simulink model "magnetorquer"  (R2019b)
settings: Solver=VariableStepAuto  StartTime=0.0  StopTime=10.0  RelTol=1e-3
libraries: vrlib x1
settings Model: Creator=Florian  LastModifiedBy=robin

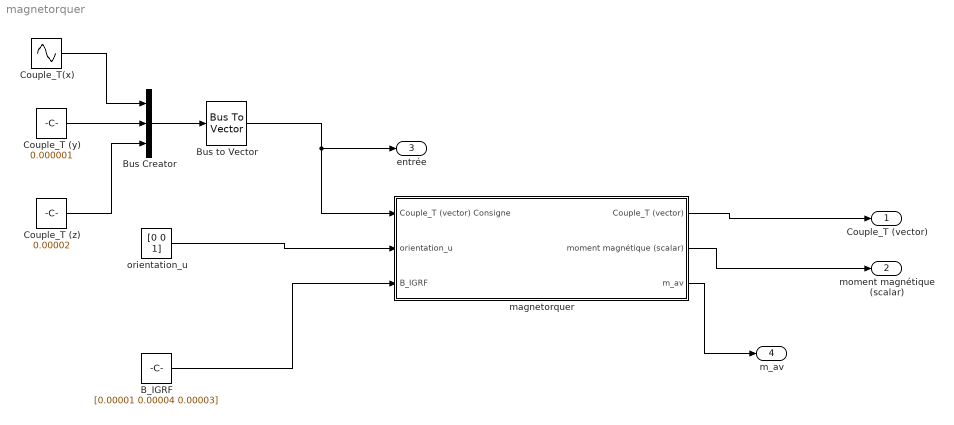
== system magnetorquer ==
  B_IGRF : Constant  Value=[0.00001 0.00004 0.00003]
  Bus Creator : BusCreator  Inputs=3
  Bus to Vector : BusToVector
  Couple_T (y) : Constant  Value=0.000001
  "Couple_T (z) " : Constant  Value=0.00002
  Couple_T(x) : Sin  Amplitude=0.00005  Phase=0.2  SampleTime=0
  magnetorquer : Subsystem
  "orientation_u " : Constant  Value=[0 0 1]
  "Couple_T (vector) " : Outport
  moment magnétique (scalar) : Outport  Port=2
  entrée : Outport  Port=3
  m_av : Outport  Port=4
  wires:
  Bus to Vector/1 -> entrée/1, magnetorquer/1(Couple_T (vector) Consigne)
  "orientation_u "/1 -> magnetorquer/2(orientation_u)
  B_IGRF/1 -> magnetorquer/3(B_IGRF)
  magnetorquer/1("Couple_T (vector) ") -> "Couple_T (vector) "/1
  magnetorquer/2(moment magnétique (scalar)) -> moment magnétique (scalar)/1
  Bus Creator/1 -> Bus to Vector/1
  Couple_T (y)/1 -> Bus Creator/2
  "Couple_T (z) "/1 -> Bus Creator/3
  Couple_T(x)/1 -> Bus Creator/1
  magnetorquer/3(m_av) -> m_av/1

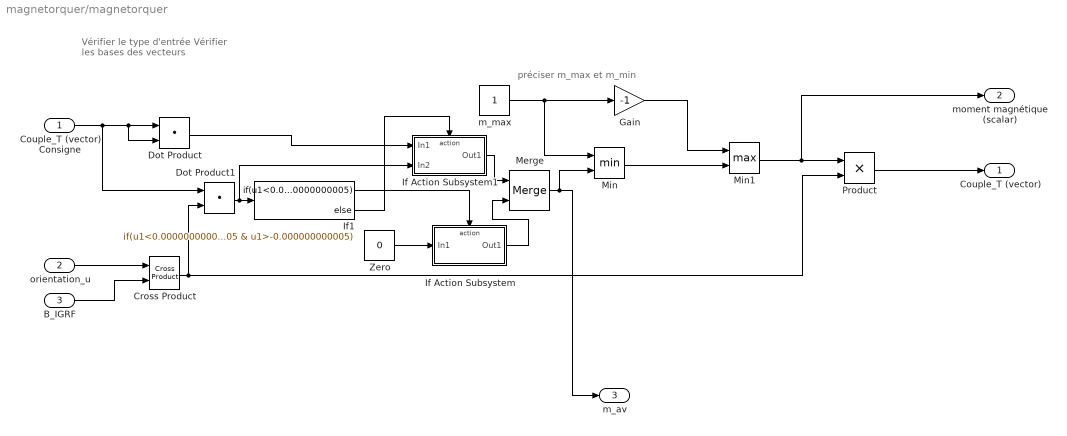
== system magnetorquer/magnetorquer ==
  note: Vérifier le type d'entrée
      | Vérifier les bases des vecteurs
  note: préciser m_max et m_min
  Couple_T (vector) Consigne : Inport  PortDimensions=3
  orientation_u : Inport  Port=2  PortDimensions=3
  B_IGRF : Inport  Port=3  PortDimensions=3
  Cross Product : vrlib/Utilities/Cross Product
      settings: SourceProductName=Simulink
  Dot Product : DotProduct  InputSameDT=on  OutDataTypeStr=Inherit: Inherit via internal rule
  Dot Product1 : DotProduct  InputSameDT=on  OutDataTypeStr=Inherit: Inherit via internal rule
  Gain : Gain  Gain=-1
  If Action Subsystem : Subsystem  TreatAsAtomicUnit=on
  If Action Subsystem1 : Subsystem  TreatAsAtomicUnit=on
  If1 : If  IfExpression=u1<0.000000000005 & u1>-0.000000000005
  Merge : Merge
  Min : MinMax  Inputs=2
  Min1 : MinMax  Function=max  Inputs=2
  Product : Product
  Zero : Constant  Value=0  OutDataTypeStr=Inherit: Inherit via back propagation
  m_max : Constant
  "Couple_T (vector) " : Outport
  moment magnétique (scalar) : Outport  Port=2
  m_av : Outport  Port=3
  wires:
  m_max/1 -> Min/1, Gain/1
  Cross Product/1 -> Product/2, Dot Product1/2
  B_IGRF/1 -> Cross Product/2
  Dot Product1/1 -> If Action Subsystem1/2(In2), If1/1
  Couple_T (vector) Consigne/1 -> Dot Product1/1, Dot Product/1, Dot Product/2
  orientation_u/1 -> Cross Product/1
  Min1/1 -> moment magnétique (scalar)/1, Product/1
  Merge/1 -> Min/2, m_av/1
  Min/1 -> Min1/2
  Gain/1 -> Min1/1
  Product/1 -> "Couple_T (vector) "/1
  If Action Subsystem1/1(Out1) -> Merge/1
  If Action Subsystem/1(Out1) -> Merge/2
  Zero/1 -> If Action Subsystem/1(In1)
  Dot Product/1 -> If Action Subsystem1/1(In1)
  If1/1 -> If Action Subsystem/Action
  If1/2 -> If Action Subsystem1/Action

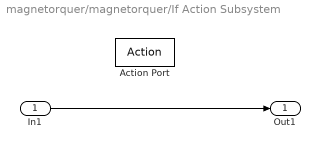
== system magnetorquer/magnetorquer/If Action Subsystem ==
  In1 : Inport
  Action Port : ActionPort  ActionPortLabel=if(u1<0.000000000005 & u1>-0.000000000005)
  Out1 : Outport
  wires:
  In1/1 -> Out1/1

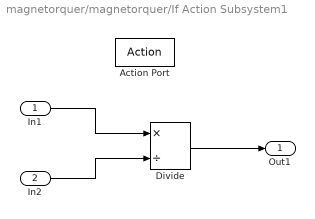
== system magnetorquer/magnetorquer/If Action Subsystem1 ==
  In1 : Inport
  In2 : Inport  Port=2
  Action Port : ActionPort  ActionPortLabel=else
  Divide : Product  Inputs=*/
  Out1 : Outport
  wires:
  In1/1 -> Divide/1
  In2/1 -> Divide/2
  Divide/1 -> Out1/1
